simulink model "HydroPowertest"  (R2024b)
settings: Solver=FixedStepAuto  StartTime=0.0  StopTime=10  FixedStep=0.0001  RelTol=1e-3
values from neighbouring files (symbols this model uses):
  A = [0 Lq 0;-Ld 0 Mf]    [Generator_Datatest.m]
  Acc = [0 Lq 0;-Ld 0 Mf;0 0 0]    [Generator_Datatest.m]
  Af = 0.01    [Data__MOTOR.m]    (also in Generator_Data.m = 0.0001; Generator_Datatest.m)
  Bf = 0.0002    [Data__MOTOR.m]    (also in Generator_Data.m = 2e-05; Generator_Datatest.m)
  Cc = Cc0+6*Cc0    (= 0.7)    [Data__MOTOR.m]    (also in Generator_Datatest.m)
  Cc0 = 0.1    [Data__MOTOR.m]    (also in Generator_Datatest.m)
  CurrentFaultSwitch = 0    [Data__MOTOR.m]    (also in Generator_Data.m = 1; Generator_Datatest.m)
  Jm = 0.08    [Data__MOTOR.m]    (also in Generator_Datatest.m)
  Ke = 0.139    [Data__MOTOR.m]    (also in Generator_Datatest.m)
  Lcc = [-Ld 0 Mf;0 -Lq 0;-Mf 0 Lf]    [Generator_Datatest.m]
  Le = 0.44    [Data__MOTOR.m]    (also in Generator_Datatest.m)
  Lf = 0.0924    [Generator_Datatest.m]
  P = 4    [Generator_Data.m]    (also in Generator_Datatest.m = 3)
  R = 42.3    [Data__MOTOR.m]    (also in Generator_Datatest.m = [Rs 0 0;0 Rs 0])
  rate_noise_i = 0.02*In    (= 0.22)    [Data__MOTOR.m]    (also in Generator_Data.m = 0.02; Generator_Datatest.m)
  rate_noise_w = 0.02*Wn    (= 2.96)    [Data__MOTOR.m]    (also in Generator_Data.m = 0.002; Generator_Datatest.m)
  Rcc = [Rs 0 0;0 Rs 0;0 0 Rf]    [Generator_Datatest.m]
  Re = 2.4    [Data__MOTOR.m]    (also in Generator_Datatest.m)
  Rf = 10    [Generator_Datatest.m]
  Rm = 0.01    [Data__MOTOR.m]    (also in Generator_Datatest.m)
  sinamp = 384.6    [Generator_Datatest.m]
  StartStop = 0    [Data__MOTOR.m]    (also in Generator_Data.m; Generator_Datatest.m)
  Te = 0.1    [Data__MOTOR.m]    (also in Generator_Data.m = 1; Generator_Datatest.m)
  Ua = 48    [Data__MOTOR.m]    (also in Generator_Datatest.m)
  VelocityFaultSwitch = 0    [Data__MOTOR.m]    (also in Generator_Data.m = 1; Generator_Datatest.m)
  Vf = 300    [Generator_Datatest.m]
undefined symbols (not defined in the file or in its folder): dspblkCoreblockFVToolHelper, gcbh, sigbuilder_block
libraries: SignalEditorBlockLib x5
(part 3 of 3)

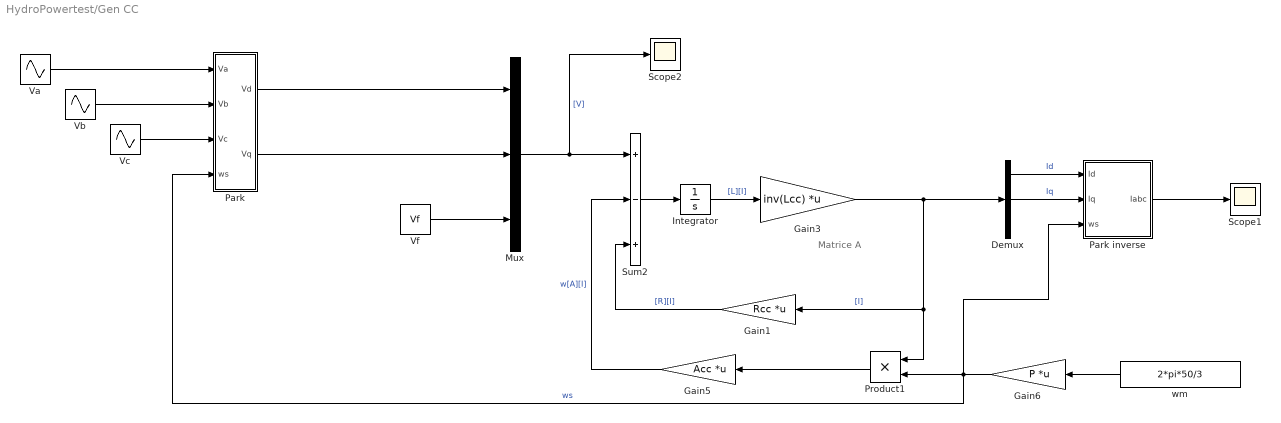
== system HydroPowertest/Gen CC ==
  note: Matrice A
  Demux : Demux  Outputs=3
  Gain1 : Gain  Gain=Rcc  Multiplication=Matrix(K*u)
  Gain3 : Gain  Gain=inv(Lcc)  Multiplication=Matrix(K*u)
  Gain5 : Gain  Gain=Acc  Multiplication=Matrix(K*u)
  Gain6 : Gain  Gain=P  Multiplication=Matrix(K*u)
  Integrator : Integrator
  Mux : Mux  Inputs=3
  Park : Subsystem
  Park inverse : Subsystem
  Product1 : Product
  Scope1 : Scope
  Scope2 : Scope
  Sum2 : Sum  Inputs=+-+
  "Va " : Sin  Amplitude=sinamp  Frequency=50*2*pi  SampleTime=0
  "Vb " : Sin  Amplitude=sinamp  Frequency=50*2*pi  Phase=-2*pi/3  SampleTime=0
  Vc : Sin  Amplitude=sinamp  Frequency=50*2*pi  Phase=2*pi/3  SampleTime=0
  Vf : Constant  Value=Vf
  wm : Constant  Value=2*pi*50/3
  wires:
  Park/2(Vq) -> Mux/2
  Park/1(Vd) -> Mux/1
  Vf/1 -> Mux/3
  Mux/1 -> Scope2/1, Sum2/1  "[V]"
  Sum2/1 -> Integrator/1
  Integrator/1 -> Gain3/1  "[L][I]"
  Gain1/1 -> Sum2/3  "[R][I]"
  Product1/1 -> Gain5/1
  Gain5/1 -> Sum2/2  "w[A][I]"
  Demux/1 -> Park inverse/1(Id)  "Id"
  Demux/2 -> Park inverse/2(Iq)  "Iq"
  Gain3/1 -> Demux/1, Gain1/1, Product1/1  "[I]"
  Gain6/1 -> Park inverse/3(ws), Park/4(ws), Product1/2  "ws"
  wm/1 -> Gain6/1
  Park inverse/1(Iabc) -> Scope1/1
  "Va "/1 -> Park/1(Va)
  "Vb "/1 -> Park/2(Vb)
  Vc/1 -> Park/3(Vc)

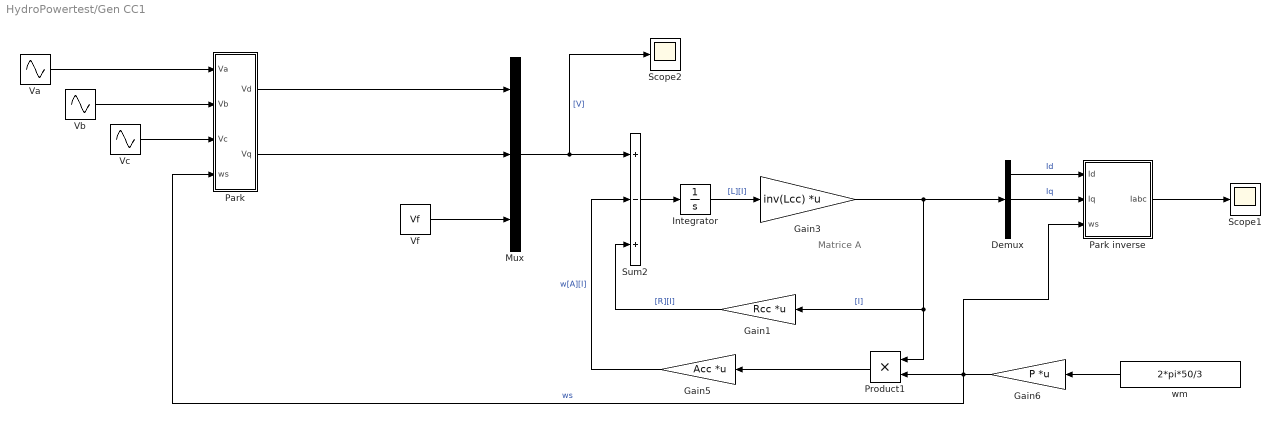
== system HydroPowertest/Gen CC1 ==
  note: Matrice A
  Demux : Demux  Outputs=3
  Gain1 : Gain  Gain=Rcc  Multiplication=Matrix(K*u)
  Gain3 : Gain  Gain=inv(Lcc)  Multiplication=Matrix(K*u)
  Gain5 : Gain  Gain=Acc  Multiplication=Matrix(K*u)
  Gain6 : Gain  Gain=P  Multiplication=Matrix(K*u)
  Integrator : Integrator
  Mux : Mux  Inputs=3
  Park : Subsystem
  Park inverse : Subsystem
  Product1 : Product
  Scope1 : Scope
  Scope2 : Scope
  Sum2 : Sum  Inputs=+-+
  "Va " : Sin  Amplitude=sinamp  Frequency=50*2*pi  SampleTime=0
  "Vb " : Sin  Amplitude=sinamp  Frequency=50*2*pi  Phase=-2*pi/3  SampleTime=0
  Vc : Sin  Amplitude=sinamp  Frequency=50*2*pi  Phase=2*pi/3  SampleTime=0
  Vf : Constant  Value=Vf
  wm : Constant  Value=2*pi*50/3
  wires:
  Vc/1 -> Park/3(Vc)
  "Vb "/1 -> Park/2(Vb)
  "Va "/1 -> Park/1(Va)
  Park inverse/1(Iabc) -> Scope1/1
  wm/1 -> Gain6/1
  Gain6/1 -> Product1/2, Park/4(ws), Park inverse/3(ws)  "ws"
  Gain3/1 -> Product1/1, Gain1/1, Demux/1  "[I]"
  Demux/2 -> Park inverse/2(Iq)  "Iq"
  Demux/1 -> Park inverse/1(Id)  "Id"
  Gain5/1 -> Sum2/2  "w[A][I]"
  Product1/1 -> Gain5/1
  Gain1/1 -> Sum2/3  "[R][I]"
  Integrator/1 -> Gain3/1  "[L][I]"
  Sum2/1 -> Integrator/1
  Mux/1 -> Sum2/1, Scope2/1  "[V]"
  Vf/1 -> Mux/3
  Park/1(Vd) -> Mux/1
  Park/2(Vq) -> Mux/2

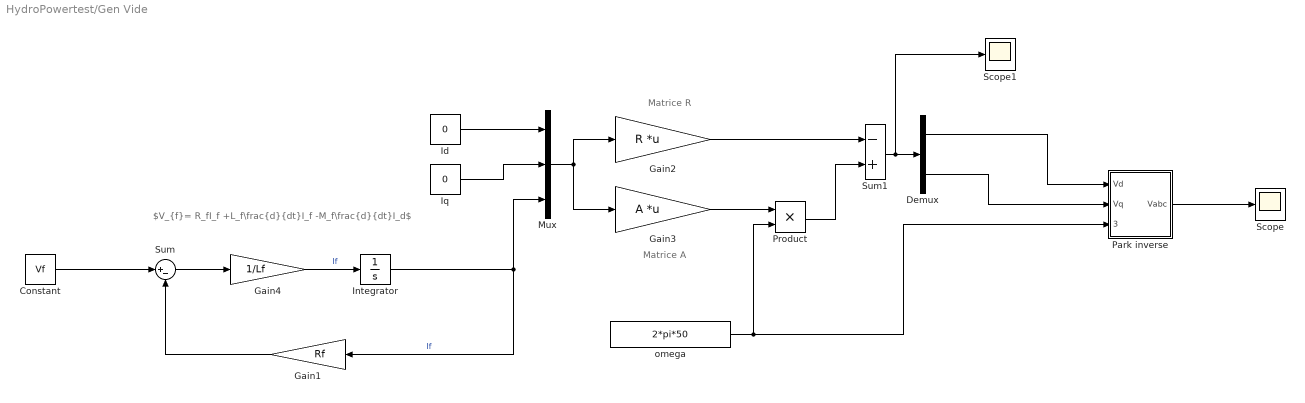
== system HydroPowertest/Gen Vide ==
  note: Matrice R
  note: $V_{f}= R_fI_f +L_f\frac{d}{dt}I_f -M_f\frac{d}{dt}I_d$
  note: Matrice A
  Constant : Constant  Value=Vf
  Demux : Demux  Outputs=2
  Gain1 : Gain  Gain=Rf
  Gain2 : Gain  Gain=R  Multiplication=Matrix(K*u)
  Gain3 : Gain  Gain=A  Multiplication=Matrix(K*u)
  Gain4 : Gain  Gain=1/Lf
  Id : Constant  Value=0
  Integrator : Integrator
  Iq : Constant  Value=0
  Mux : Mux  Inputs=3
  Park inverse : Subsystem
  Product : Product
  Scope : Scope
  Scope1 : Scope
  Sum : Sum  Inputs=|+-
  Sum1 : Sum  Inputs=-+
  omega : Constant  Value=2*pi*50
  wires:
  Integrator/1 -> Mux/3, Gain1/1  "If"
  Constant/1 -> Sum/1
  Gain1/1 -> Sum/2
  Id/1 -> Mux/1
  Iq/1 -> Mux/2
  Gain2/1 -> Sum1/1
  Mux/1 -> Gain3/1, Gain2/1
  Gain3/1 -> Product/1
  Product/1 -> Sum1/2
  omega/1 -> Park inverse/3(omega), Product/2
  Sum1/1 -> Scope1/1, Demux/1
  Demux/1 -> Park inverse/1(Vd)
  Demux/2 -> Park inverse/2(Vq)
  Park inverse/1(Vabc) -> Scope/1
  Sum/1 -> Gain4/1
  Gain4/1 -> Integrator/1  "If"

== system HydroPowertest/HOME ==

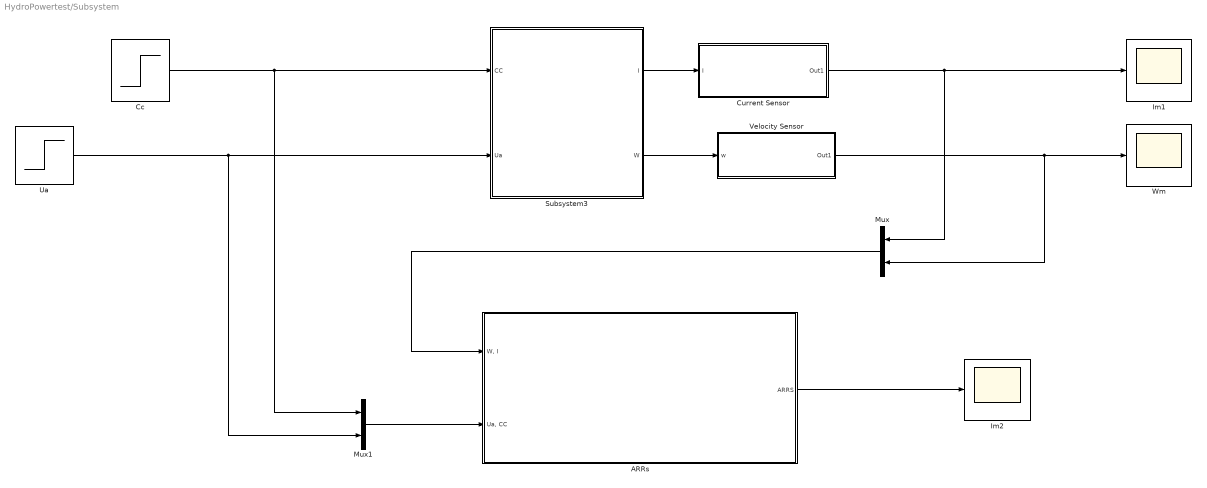
== system HydroPowertest/Subsystem ==
  ARRs : Subsystem
      mask Display: disp('ALGORITHME DE DIAGNOSTIC')
  Cc : Step  Time=30  Before=Cc0  After=Cc  SampleTime=0
  Current Sensor : Subsystem
      mask Display: disp('Current\n sensor')
  Im1 : Scope
  Im2 : Scope
  Mux : Mux  Inputs=2
  Mux1 : Mux  Inputs=2
  Subsystem3 : Subsystem
  Ua : Step  Time=0  After=Ua  SampleTime=0
  Velocity Sensor : Subsystem
      mask Display: disp('Velocity \n Sensor')
  Wm : Scope
  wires:
  Current Sensor/1(Out1) -> Mux/1, Im1/1
  Mux1/1 -> ARRs/2("Ua, CC")
  Cc/1 -> Mux1/1, Subsystem3/1(CC)
  Ua/1 -> Mux1/2, Subsystem3/2(Ua)
  Mux/1 -> ARRs/1("W, I")
  Subsystem3/1(I) -> Current Sensor/1(I)
  Subsystem3/2(W) -> Velocity Sensor/1(w)
  ARRs/1(ARRS) -> Im2/1
  Velocity Sensor/1(Out1) -> Wm/1, Mux/2

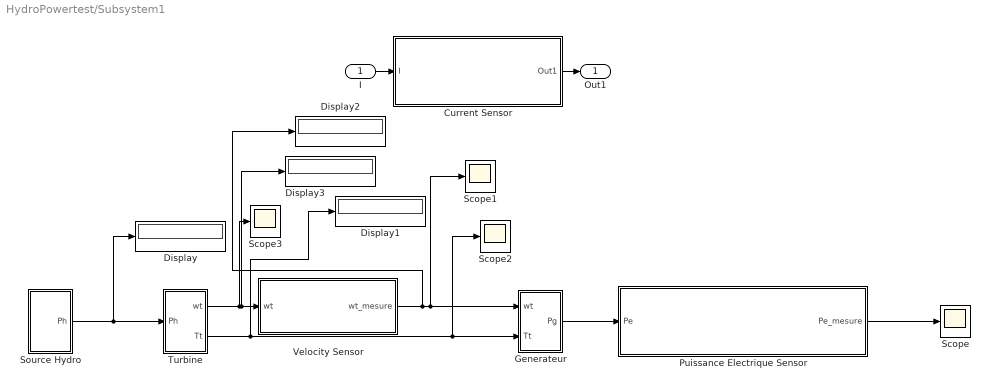
== system HydroPowertest/Subsystem1 ==
  I : Inport
  Current Sensor : Subsystem
      mask Display: disp('Current\n sensor')
  Display{,1..3} (4 alike) : Display
  Generateur : Subsystem
  Puissance Electrique Sensor : Subsystem
      mask Display: disp('Puissance Electrique\n sensor')
  Scope{,1..3} (4 alike) : Scope
  Source Hydro : Subsystem
  Turbine : Subsystem
  Velocity Sensor : Subsystem
      mask Display: disp('Velocity \n Sensor')
  Out1 : Outport
  wires:
  I/1 -> Current Sensor/1(I)
  Turbine/1(wt) -> Display3/1, Velocity Sensor/1(wt), Scope3/1
  Source Hydro/1(Ph) -> Display/1, Turbine/1(Ph)
  Turbine/2(Tt) -> Scope2/1, Generateur/2(Tt), Display1/1
  Generateur/1(Pg) -> Puissance Electrique Sensor/1(Pe)
  Current Sensor/1(Out1) -> Out1/1
  Velocity Sensor/1(wt_mesure) -> Display2/1, Scope1/1, Generateur/1(wt)
  Puissance Electrique Sensor/1(Pe_mesure) -> Scope/1

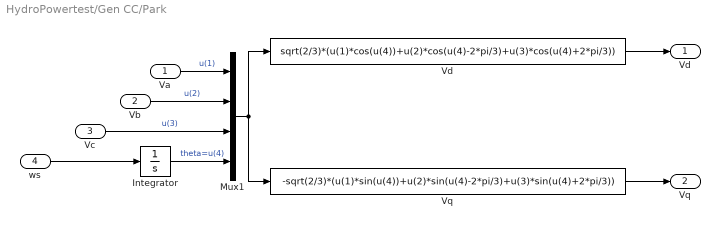
== system HydroPowertest/Gen CC/Park ==
  Va : Inport
  Vb : Inport  Port=2
  Vc : Inport  Port=3
  ws : Inport  Port=4
  Integrator : Integrator
  Mux1 : Mux
  "Vd " : Fcn  Expr=sqrt(2/3)*(u(1)*cos(u(4))+u(2)*cos(u(4)-2*pi/3)+u(3)*cos(u(4)+2*pi/3))
  "Vq " : Fcn  Expr=-sqrt(2/3)*(u(1)*sin(u(4))+u(2)*sin(u(4)-2*pi/3)+u(3)*sin(u(4)+2*pi/3))
  Vd : Outport
  Vq : Outport  Port=2
  wires:
  Mux1/1 -> "Vq "/1, "Vd "/1
  "Vd "/1 -> Vd/1
  Vb/1 -> Mux1/2  "u(2)"
  Va/1 -> Mux1/1  "u(1)"
  Integrator/1 -> Mux1/4  "theta=u(4)"
  ws/1 -> Integrator/1
  Vc/1 -> Mux1/3  "u(3)"
  "Vq "/1 -> Vq/1

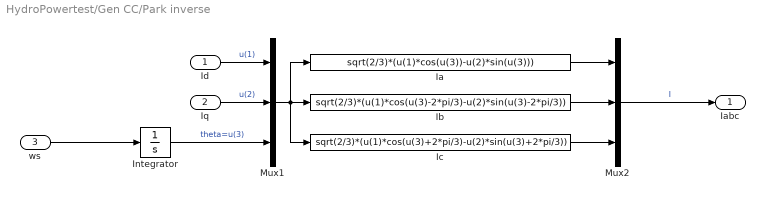
== system HydroPowertest/Gen CC/Park inverse ==
  Id : Inport
  Iq : Inport  Port=2
  ws : Inport  Port=3
  Ia : Fcn  Expr=sqrt(2/3)*(u(1)*cos(u(3))-u(2)*sin(u(3)))
  Ib : Fcn  Expr=sqrt(2/3)*(u(1)*cos(u(3)-2*pi/3)-u(2)*sin(u(3)-2*pi/3))
  Ic : Fcn  Expr=sqrt(2/3)*(u(1)*cos(u(3)+2*pi/3)-u(2)*sin(u(3)+2*pi/3))
  Integrator : Integrator
  Mux1 : Mux  Inputs=3
  Mux2 : Mux  Inputs=3
  Iabc : Outport
  wires:
  ws/1 -> Integrator/1
  Integrator/1 -> Mux1/3  "theta=u(3)"
  Id/1 -> Mux1/1  "u(1)"
  Iq/1 -> Mux1/2  "u(2)"
  Ia/1 -> Mux2/1
  Ic/1 -> Mux2/3
  Ib/1 -> Mux2/2
  Mux2/1 -> Iabc/1  "I"
  Mux1/1 -> Ia/1, Ic/1, Ib/1

== system HydroPowertest/Gen CC1/Park ==
  Va : Inport
  Vb : Inport  Port=2
  Vc : Inport  Port=3
  ws : Inport  Port=4
  Integrator : Integrator
  Mux1 : Mux
  "Vd " : Fcn  Expr=sqrt(2/3)*(u(1)*cos(u(4))+u(2)*cos(u(4)-2*pi/3)+u(3)*cos(u(4)+2*pi/3))
  "Vq " : Fcn  Expr=-sqrt(2/3)*(u(1)*sin(u(4))+u(2)*sin(u(4)-2*pi/3)+u(3)*sin(u(4)+2*pi/3))
  Vd : Outport
  Vq : Outport  Port=2
  wires:
  "Vq "/1 -> Vq/1
  Vc/1 -> Mux1/3  "u(3)"
  ws/1 -> Integrator/1
  Integrator/1 -> Mux1/4  "theta=u(4)"
  Va/1 -> Mux1/1  "u(1)"
  Vb/1 -> Mux1/2  "u(2)"
  "Vd "/1 -> Vd/1
  Mux1/1 -> "Vd "/1, "Vq "/1

== system HydroPowertest/Gen CC1/Park inverse ==
  Id : Inport
  Iq : Inport  Port=2
  ws : Inport  Port=3
  Ia : Fcn  Expr=sqrt(2/3)*(u(1)*cos(u(3))-u(2)*sin(u(3)))
  Ib : Fcn  Expr=sqrt(2/3)*(u(1)*cos(u(3)-2*pi/3)-u(2)*sin(u(3)-2*pi/3))
  Ic : Fcn  Expr=sqrt(2/3)*(u(1)*cos(u(3)+2*pi/3)-u(2)*sin(u(3)+2*pi/3))
  Integrator : Integrator
  Mux1 : Mux  Inputs=3
  Mux2 : Mux  Inputs=3
  Iabc : Outport
  wires:
  Mux1/1 -> Ib/1, Ic/1, Ia/1
  Mux2/1 -> Iabc/1  "I"
  Ib/1 -> Mux2/2
  Ic/1 -> Mux2/3
  Ia/1 -> Mux2/1
  Iq/1 -> Mux1/2  "u(2)"
  Id/1 -> Mux1/1  "u(1)"
  Integrator/1 -> Mux1/3  "theta=u(3)"
  ws/1 -> Integrator/1

== system HydroPowertest/Gen Vide/Park inverse ==
  Vd : Inport
  Vq : Inport  Port=2
  omega : Inport  Port=3
  Integrator : Integrator
  Mux1 : Mux  Inputs=3
  Mux2 : Mux  Inputs=3
  Va : Fcn  Expr=sqrt(2/3)*(u(1)*cos(u(3))-u(2)*sin(u(3)))
  Vb : Fcn  Expr=sqrt(2/3)*(u(1)*cos(u(3)-2*pi/3)-u(2)*sin(u(3)-2*pi/3))
  Vc : Fcn  Expr=sqrt(2/3)*(u(1)*cos(u(3)+2*pi/3)-u(2)*sin(u(3)+2*pi/3))
  Vabc : Outport
  wires:
  Mux1/1 -> Vc/1, Vb/1, Va/1
  Mux2/1 -> Vabc/1  "V"
  Vb/1 -> Mux2/2
  Vc/1 -> Mux2/3
  Va/1 -> Mux2/1
  Vq/1 -> Mux1/2
  Vd/1 -> Mux1/1
  Integrator/1 -> Mux1/3  "theta"
  omega/1 -> Integrator/1

== system HydroPowertest/Subsystem/ARRs ==
  "W, I" : Inport
  "Ua, CC" : Inport  Port=2
  ARR1 : Subsystem
      mask Display: disp('Residu 1')
  ARR2 : Subsystem
      mask Display: disp('Residu 2')
  Demux : Demux  Outputs=2
  Demux1 : Demux  Outputs=2
  Mux : Mux  Inputs=2
  Scope : Scope
  ARRS : Outport  VectorParamsAs1DForOutWhenUnconnected=off
  wires:
  "W, I"/1 -> Demux1/1
  Demux/1 -> ARR1/1(Im1), ARR2/1(Im1)
  Demux/2 -> ARR2/2(Wm), ARR1/2(Wm)
  "Ua, CC"/1 -> Demux/1
  Demux1/1 -> ARR1/3(" Ua")
  Demux1/2 -> ARR2/3(CC: Couple de charge)
  ARR1/1(R1) -> Mux/1
  ARR2/1(r2) -> Scope/1, Mux/2
  Mux/1 -> ARRS/1

== system HydroPowertest/Subsystem/Current Sensor ==
  I : Inport
  CurrentFaultSwitch : Constant  Value=CurrentFaultSwitch
  Dot Product : DotProduct  OutDataTypeStr=Inherit: Inherit via internal rule
  Noise1 : UniformRandomNumber  Minimum=-rate_noise_i  Maximum=+rate_noise_i  SampleTime=0.1
  Scope : Scope
  Signal Editor : SignalEditorBlockLib/Signal Editor  FileName=CurrentFault.mat  ActiveScenario=ChuteCourant  ActiveSignal=Fault  IsBus=off  OutputBusObjectStr=Bus: BusObject  SampleTime=0  Interpolate=off  ZeroCross=off  OutputAfterFinalValue=Setting to zero  Unit=inherit  PreserveSignalName=on  ApplySigPropsToAllScenarios=on  ApplySigPropsToAllSignals=off
  Sum3 : Sum  InputSameDT=on  SaturateOnIntegerOverflow=on  OutDataTypeStr=Inherit: Same as first input
  Switch : Switch  Criteria=u2 > Threshold  SaturateOnIntegerOverflow=off  InputSameDT=off
  Out1 : Outport  VectorParamsAs1DForOutWhenUnconnected=off
  wires:
  Sum3/1 -> Out1/1
  Noise1/1 -> Sum3/2
  Dot Product/1 -> Switch/1
  I/1 -> Switch/3, Dot Product/2
  Signal Editor/1 -> Dot Product/1
  Switch/1 -> Sum3/1, Scope/1
  CurrentFaultSwitch/1 -> Switch/2

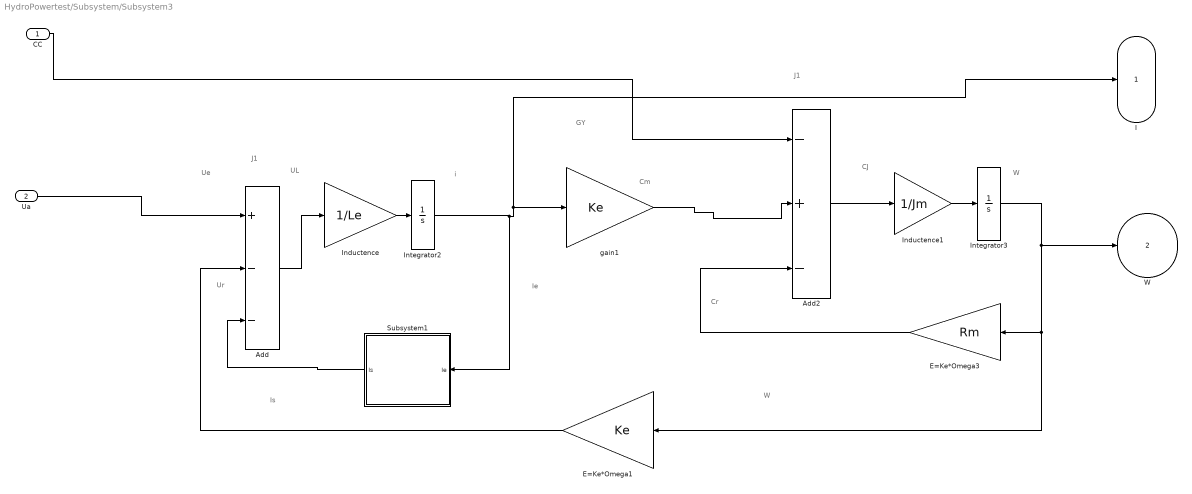
== system HydroPowertest/Subsystem/Subsystem3 ==
  note: J1
  note: i
  note: GY
  note: J1
  note: UL
  note: Ue
  note: Cr
  note: W
  note: Cm
  note: CJ
  note: Ur
  note: W
  note: Is
  note: Ie
  CC : Inport
  Ua : Inport  Port=2
  Add : Sum  Inputs=+--
  Add2 : Sum  Inputs=-+-
  E=Ke*Omega1 : Gain  Gain=Ke
  E=Ke*Omega3 : Gain  Gain=Rm
  Inductence : Gain  Gain=1/Le
  Inductence1 : Gain  Gain=1/Jm
  Integrator2 : Integrator
  Integrator3 : Integrator
  Subsystem1 : Subsystem
      mask Display: disp('Re')
  gain1 : Gain  Gain=Ke
  I : Outport
  W : Outport  Port=2
  wires:
  E=Ke*Omega3/1 -> Add2/3
  gain1/1 -> Add2/2
  Integrator3/1 -> E=Ke*Omega3/1, E=Ke*Omega1/1, W/1
  Ua/1 -> Add/1
  Integrator2/1 -> Subsystem1/1(Ie), I/1, gain1/1
  Subsystem1/1(Is) -> Add/3
  Inductence/1 -> Integrator2/1
  Add2/1 -> Inductence1/1
  Add/1 -> Inductence/1
  Inductence1/1 -> Integrator3/1
  E=Ke*Omega1/1 -> Add/2
  CC/1 -> Add2/1

== system HydroPowertest/Subsystem/Velocity Sensor ==
  note: I
  w : Inport
  Dot Product : DotProduct  OutDataTypeStr=Inherit: Inherit via internal rule
  Noise1 : UniformRandomNumber  Minimum=-rate_noise_w  Maximum=+rate_noise_w  SampleTime=0.1
  Signal Editor : SignalEditorBlockLib/Signal Editor  FileName=VelocityFault.mat  ActiveScenario=ChuteVelocite  ActiveSignal=Fault  IsBus=off  OutputBusObjectStr=Bus: BusObject  SampleTime=0  Interpolate=off  ZeroCross=off  OutputAfterFinalValue=Setting to zero  Unit=inherit  PreserveSignalName=on  ApplySigPropsToAllScenarios=on  ApplySigPropsToAllSignals=off
  Sum3 : Sum  InputSameDT=on  SaturateOnIntegerOverflow=on  OutDataTypeStr=Inherit: Same as first input
  Velocity Sensor Switch : Switch  Criteria=u2 ~= 0  Threshold=1  SaturateOnIntegerOverflow=off  InputSameDT=off
  VelocityFaultSwitch : Constant  Value=VelocityFaultSwitch
  Out1 : Outport  VectorParamsAs1DForOutWhenUnconnected=off
  wires:
  Sum3/1 -> Out1/1
  w/1 -> Dot Product/2, Velocity Sensor Switch/3
  Signal Editor/1 -> Dot Product/1
  Dot Product/1 -> Velocity Sensor Switch/1
  Velocity Sensor Switch/1 -> Sum3/2
  Noise1/1 -> Sum3/1
  VelocityFaultSwitch/1 -> Velocity Sensor Switch/2

== system HydroPowertest/Subsystem1/Current Sensor ==
  I : Inport
  CurrentFaultSwitch : Constant  Value=CurrentFaultSwitch
  Dot Product : DotProduct  OutDataTypeStr=Inherit: Inherit via internal rule
  Noise1 : UniformRandomNumber  Minimum=-rate_noise_i  Maximum=+rate_noise_i  SampleTime=0.1
  Scope : Scope
  Signal Editor : SignalEditorBlockLib/Signal Editor  FileName=CurrentFault.mat  ActiveScenario=ChuteCourant  ActiveSignal=Fault  IsBus=off  OutputBusObjectStr=Bus: BusObject  SampleTime=0  Interpolate=off  ZeroCross=off  OutputAfterFinalValue=Setting to zero  Unit=inherit  PreserveSignalName=on  ApplySigPropsToAllScenarios=on  ApplySigPropsToAllSignals=off
  Sum3 : Sum  InputSameDT=on  SaturateOnIntegerOverflow=on  OutDataTypeStr=Inherit: Same as first input
  Switch : Switch  Criteria=u2 > Threshold  SaturateOnIntegerOverflow=off  InputSameDT=off
  Out1 : Outport  VectorParamsAs1DForOutWhenUnconnected=off
  wires:
  Sum3/1 -> Out1/1
  Noise1/1 -> Sum3/2
  Dot Product/1 -> Switch/1
  I/1 -> Switch/3, Dot Product/2
  Signal Editor/1 -> Dot Product/1
  Switch/1 -> Sum3/1, Scope/1
  CurrentFaultSwitch/1 -> Switch/2

== system HydroPowertest/Subsystem1/Generateur ==
  wt : Inport
  Tt : Inport  Port=2
  Product1 : Product  Inputs=3
  n : Constant  Value=0.92
  Pg : Outport
  wires:
  n/1 -> Product1/1
  Tt/1 -> Product1/3
  wt/1 -> Product1/2
  Product1/1 -> Pg/1

== system HydroPowertest/Subsystem1/Puissance Electrique Sensor ==
  Pe : Inport
  CurrentFaultSwitch : Constant  Value=CurrentFaultSwitch
  Dot Product : DotProduct  OutDataTypeStr=Inherit: Inherit via internal rule
  Noise1 : UniformRandomNumber  Minimum=-rate_noise_i  Maximum=+rate_noise_i  SampleTime=0.1
  Scope : Scope
  Signal Editor : SignalEditorBlockLib/Signal Editor  FileName=CurrentFault.mat  ActiveScenario=ChuteCourant  ActiveSignal=Fault  IsBus=off  OutputBusObjectStr=Bus: BusObject  SampleTime=0  Interpolate=off  ZeroCross=off  OutputAfterFinalValue=Setting to zero  Unit=inherit  PreserveSignalName=on  ApplySigPropsToAllScenarios=on  ApplySigPropsToAllSignals=off
  Sum3 : Sum  InputSameDT=on  SaturateOnIntegerOverflow=on  OutDataTypeStr=Inherit: Same as first input
  Switch : Switch  Criteria=u2 > Threshold  SaturateOnIntegerOverflow=off  InputSameDT=off
  Pe_mesure : Outport  VectorParamsAs1DForOutWhenUnconnected=off
  wires:
  CurrentFaultSwitch/1 -> Switch/2
  Switch/1 -> Scope/1, Sum3/1
  Signal Editor/1 -> Dot Product/1
  Pe/1 -> Dot Product/2, Switch/3
  Dot Product/1 -> Switch/1
  Noise1/1 -> Sum3/2
  Sum3/1 -> Pe_mesure/1

== system HydroPowertest/Subsystem1/Source Hydro ==
  H : Constant  Value=50
  Puissance Hydro : Product  Inputs=4
  Q : Constant  Value=20
  g : Constant  Value=9.81
  rho : Constant  Value=1000
  Ph : Outport
  wires:
  Q/1 -> Puissance Hydro/3
  g/1 -> Puissance Hydro/2
  H/1 -> Puissance Hydro/4
  Puissance Hydro/1 -> Ph/1
  rho/1 -> Puissance Hydro/1

== system HydroPowertest/Subsystem1/Turbine ==
  Ph : Inport
  Gain : Gain  Gain=0.85
  Integrator : Integrator
  wt : Outport
  Tt : Outport  Port=2
  wires:
  Gain/1 -> Tt/1, Integrator/1
  Ph/1 -> Gain/1
  Integrator/1 -> wt/1

== system HydroPowertest/Subsystem1/Velocity Sensor ==
  wt : Inport
  Dot Product : DotProduct  OutDataTypeStr=Inherit: Inherit via internal rule
  Noise1 : UniformRandomNumber  Minimum=-rate_noise_w  Maximum=+rate_noise_w  SampleTime=0.1
  Signal Editor : SignalEditorBlockLib/Signal Editor  FileName=VelocityFault.mat  ActiveScenario=ChuteVelocite  ActiveSignal=Fault  IsBus=off  OutputBusObjectStr=Bus: BusObject  SampleTime=0  Interpolate=off  ZeroCross=off  OutputAfterFinalValue=Setting to zero  Unit=inherit  PreserveSignalName=on  ApplySigPropsToAllScenarios=on  ApplySigPropsToAllSignals=off
  Sum3 : Sum  InputSameDT=on  SaturateOnIntegerOverflow=on  OutDataTypeStr=Inherit: Same as first input
  Velocity Sensor Switch : Switch  Criteria=u2 ~= 0  Threshold=1  SaturateOnIntegerOverflow=off  InputSameDT=off
  VelocityFaultSwitch : Constant  Value=VelocityFaultSwitch
  wt_mesure : Outport  VectorParamsAs1DForOutWhenUnconnected=off
  wires:
  Sum3/1 -> wt_mesure/1
  wt/1 -> Dot Product/2, Velocity Sensor Switch/3
  Signal Editor/1 -> Dot Product/1
  Dot Product/1 -> Velocity Sensor Switch/1
  Velocity Sensor Switch/1 -> Sum3/2
  Noise1/1 -> Sum3/1
  VelocityFaultSwitch/1 -> Velocity Sensor Switch/2

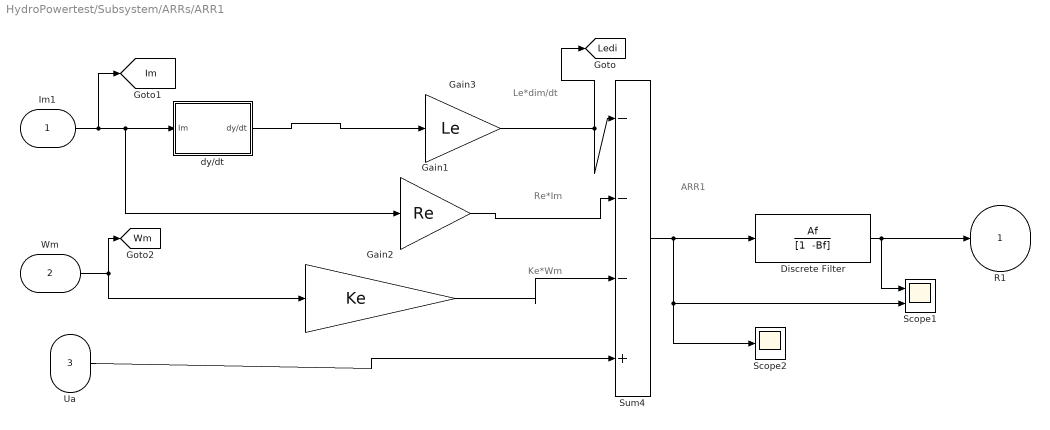
== system HydroPowertest/Subsystem/ARRs/ARR1 ==
  note: ARR1
  note: Re*Im
  note: Le*dim/dt
  note: Ke*Wm
  Im1 : Inport
  Wm : Inport  Port=2
  " Ua" : Inport  Port=3
  Discrete Filter : DiscreteFilter  LoadFcn=dspblkCoreblockFVToolHelper(gcbh,'load');  Numerator=Af  Denominator="[1  -Bf]"  SampleTime=Te  a0EqualsOne=on
      settings: CopyFcn=dspblkCoreblockFVToolHelper(gcbh,'copy');  DeleteFcn=dspblkCoreblockFVToolHelper(gcbh,'close');  ModelCloseFcn=dspblkCoreblockFVToolHelper(gcbh,'close');  PreSaveFcn=dspblkCoreblockFVToolHelper(gcbh,'presave');  PostSaveFcn=dspblkCoreblockFVToolHelper(gcbh,'postsave');  CloseFcn=dspblkCoreblockFVToolHelper(gcbh,'close');
  Gain1 : Gain  Gain=Re
  Gain2 : Gain  Gain=Ke
  Gain3 : Gain  Gain=Le
  Scope1 : Scope  NumInputPorts=2
  Scope2 : Scope
  Sum4 : Sum  Inputs=|---+
  dy/dt : Subsystem
  R1 : Outport  VectorParamsAs1DForOutWhenUnconnected=off
  tag scope: Im=global, Ledi=global, Wm=global
  wires:
  Gain1/1 -> Sum4/2
  Wm/1 -> [Wm], Gain2/1
  Gain2/1 -> Sum4/3
  " Ua"/1 -> Sum4/4
  Im1/1 -> [Im], dy/dt/1(Im), Gain1/1
  Gain3/1 -> [Ledi], Sum4/1
  dy/dt/1(dy/dt) -> Gain3/1
  Sum4/1 -> Discrete Filter/1, Scope1/2, Scope2/1
  Discrete Filter/1 -> R1/1, Scope1/1

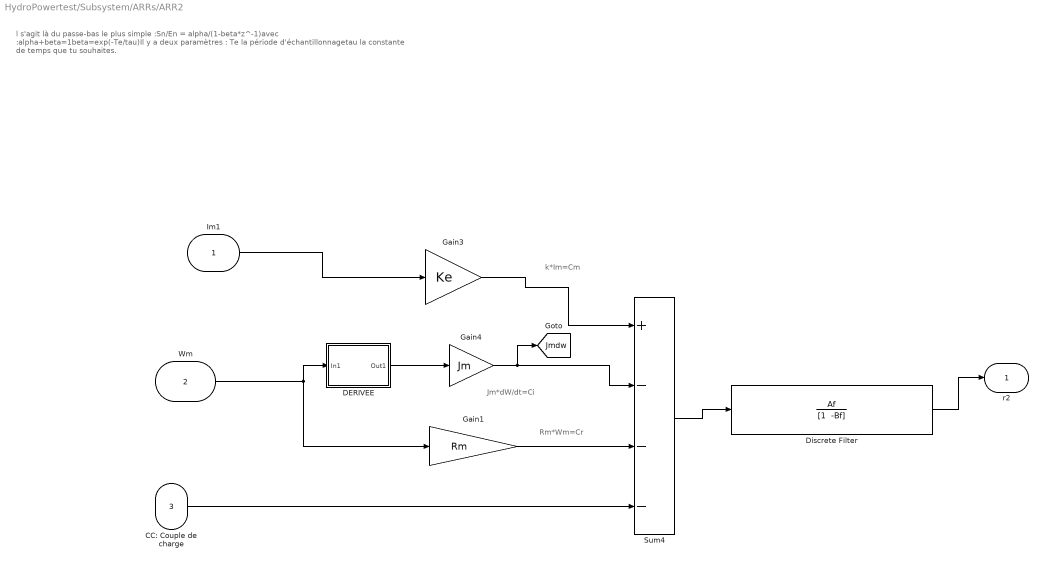
== system HydroPowertest/Subsystem/ARRs/ARR2 ==
  note: l s'agit là du passe-bas le plus simple :Sn/En = alpha/(1-beta*z^-1)avec :alpha+beta=1beta=exp(-Te/tau)Il y a deux paramètres : Te la période d'échantillonnagetau la constante de temps que tu souhaites.
  note: Rm*Wm=Cr
  note: k*Im=Cm
  note: Jm*dW/dt=Ci
  Im1 : Inport
  Wm : Inport  Port=2
  CC: Couple de charge : Inport  Port=3
  DERIVEE : Subsystem
  Discrete Filter : DiscreteFilter  Numerator=Af  Denominator="[1  -Bf]"  SampleTime=Te  a0EqualsOne=on
  Gain1 : Gain  Gain=Rm
  Gain3 : Gain  Gain=Ke
  Gain4 : Gain  Gain=Jm
  Sum4 : Sum  Inputs=+---
  r2 : Outport  VectorParamsAs1DForOutWhenUnconnected=off
  tag scope: Jmdw=global
  wires:
  Im1/1 -> Gain3/1
  Gain4/1 -> [Jmdw], Sum4/2
  CC: Couple de charge/1 -> Sum4/4
  Gain1/1 -> Sum4/3
  Wm/1 -> Gain1/1, DERIVEE/1(In1)
  Sum4/1 -> Discrete Filter/1
  DERIVEE/1(Out1) -> Gain4/1
  Discrete Filter/1 -> r2/1
  Gain3/1 -> Sum4/1

== system HydroPowertest/Subsystem/Subsystem3/Subsystem1 ==
  note: Re nominal
  note: R=Ren+Ren*(SigmaRe)
  Ie : Inport
  Constant1 : Constant  Value=Re
  Electr resistance fault : ManualSwitch  CurrentSetting=0
  Gain3 : Gain  Gain=Re
  Product : Product  Inputs=3
  Signal Builder : Subsystem  Tag=STV Subsys  LoadFcn=sigbuilder_block('load');  StartFcn=sigbuilder_block('start');  StopFcn=sigbuilder_block('stop');  ClipboardFcn=sigbuilder_block('clipboard');  mask(Sigbuilder block){tuvar=[0:10]}
      mask help: Simulink:masks:SigbuilderBlock_MD
      mask init:
      | if ~strcmp(get_param(bdroot(gcbh),'SimulationStatus'),'stopped') tuvar = sigbuilder_block('maskInit'); end
      settings: CopyFcn=sigbuilder_block('copy');  DeleteFcn=sigbuilder_block('delete');  ModelCloseFcn=sigbuilder_block('modelClose');  PreSaveFcn=sigbuilder_block('preSave');  PauseFcn=sigbuilder_block('pause');  ContinueFcn=sigbuilder_block('continue');  NameChangeFcn=sigbuilder_block('namechange');  OpenFcn=sigbuilder_block('open',[1280 104 1024 485.5 ]);  CloseFcn=sigbuilder_block('close');
      mask Display: plot(0, 0, 100, 100,[2, 2, 32, 32, 2], [68, 8, 8, 68, 68],[32, 2], [38, 38], [32, 19, 2],[53, 60, 44], [32, 17, 17, 2],[16, 16, 31, 31]);txt = getActiveGroup(gcbh);text(2, 100, txt,'verticalAlignment', 'top');
  Is : Outport
  wires:
  Product/1 -> Electr resistance fault/1
  Gain3/1 -> Electr resistance fault/2
  Constant1/1 -> Product/2
  Signal Builder/1(Le Fault) -> Product/1
  Ie/1 -> Gain3/1, Product/3
  Electr resistance fault/1 -> Is/1

== system HydroPowertest/Subsystem/ARRs/ARR1/dy//dt ==
  note: dY/dt= ((y(k)-y(k-1))/Te
  note: Y(k)
  note: Y(k-1
  Im : Inport
  Delay : Delay  DelayLength=1  SampleTime=Te
  Gain2 : Gain  Gain=1/Te
  Sum1 : Sum  Inputs=+-
  dy/dt : Outport  VectorParamsAs1DForOutWhenUnconnected=off
  wires:
  Gain2/1 -> dy/dt/1
  Sum1/1 -> Gain2/1
  Delay/1 -> Sum1/2
  Im/1 -> Delay/1, Sum1/1

== system HydroPowertest/Subsystem/ARRs/ARR2/DERIVEE ==
  In1 : Inport
  Delay : Delay  DelayLength=1  SampleTime=Te
  Gain2 : Gain  Gain=1/Te
  Sum1 : Sum  Inputs=+-
  Out1 : Outport  VectorParamsAs1DForOutWhenUnconnected=off
  wires:
  In1/1 -> Sum1/1, Delay/1
  Delay/1 -> Sum1/2
  Sum1/1 -> Gain2/1
  Gain2/1 -> Out1/1

== system HydroPowertest/Subsystem/Subsystem3/Subsystem1/Signal Builder ==
  Demux : Demux  Tag=STV Demux  Outputs=1
      settings: DisplayOption=none
  FromWs : FromWorkspace  Tag=STV FromWs  VariableName=tuvar
      SigBuilderData=|
      | common.afterFinalStr = 'Extrapolate'
      | common.sampleTime = 0
      | dataSet.timeRange = [0 200]
      | dataSet.name = 'Group 1'
      | sbobj.Groups.Name = 'Group 1'
      | sbobj.Groups.Signals.Name = 'Le Fault'
      | sbobj.Groups.Signals.XData = [0 53.6 53.6 80.8 80.8 119.5 144 162.5 164.5 181.6 200]
      | sbobj.Groups.Signals.YData = [1 1 0.898 0.841 1 1 1 1 1 1 1]
      | sbobj.Groups.TimeRange = [0 200]
  Le Fault : Outport  Tag=STV Outport  VectorParamsAs1DForOutWhenUnconnected=off
  wires:
  FromWs/1 -> Demux/1
  Demux/1 -> Le Fault/1
